simulink model "SDM"  (R2023b)
settings: Solver=FixedStepAuto  StartTime=0.0  StopTime=1  FixedStep=1/Fs  MaxStep=1/Fs  RelTol=1e-3
values from neighbouring files (symbols this model uses):
  f = Fs/2*linspace(0,1,NFFT/2+1)    [fft_plot.m]
undefined symbols (not defined in the file or in its folder): a1, a2, AAA, b1, b2, Fs, noise_pow1, noise_pow2
libraries: simulink x2
settings Model: Creator=mp3907  LastModifiedBy=mpolj
settings SolverCC: AlgebraicLoopSolver=TrustRegion
settings DataIOCC: ReturnWorkspaceOutputs=off
settings DebuggingCC: UnconnectedInputMsg=warning  UnconnectedOutputMsg=warning  UnconnectedLineMsg=warning  ArithmeticOperatorsInVariantConditions=warning
settings ModelReferenceCC: EnableRefExpFcnMdlSchedulingChecks=on
settings SFSimCC: CustomCodeUndefinedFunction=UseInterfaceOnly

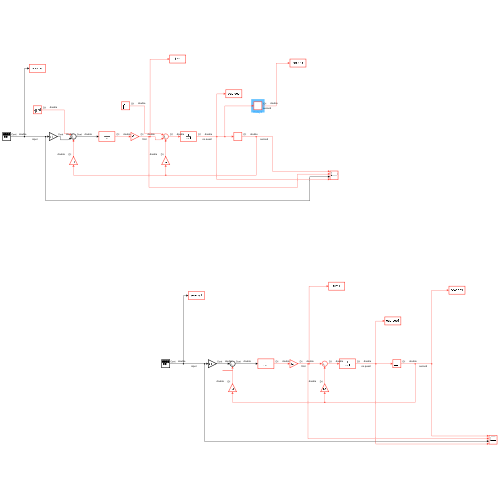
[thumbnail: Simulink's stored preview of the top-level diagram]
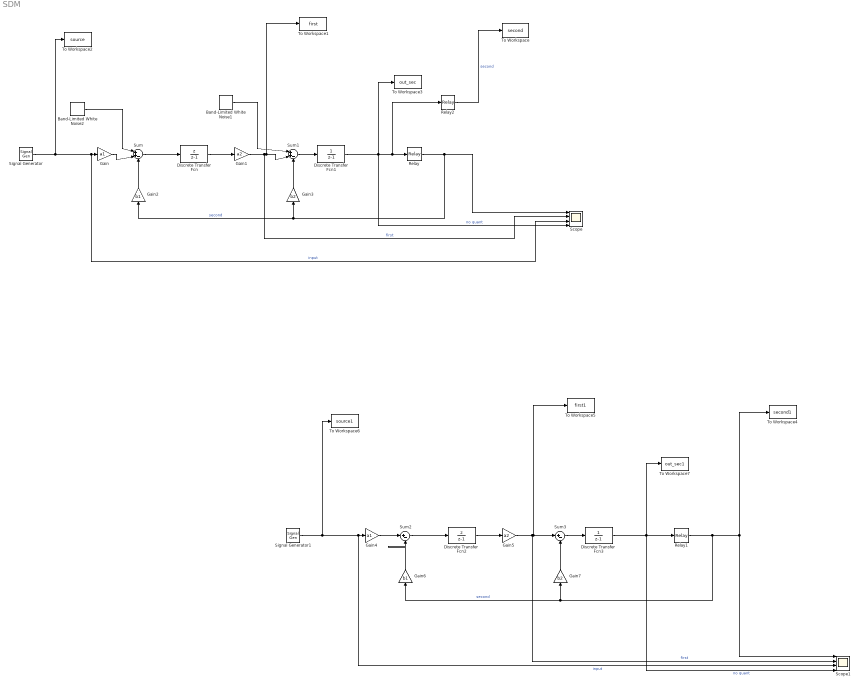
== system SDM ==
  Band-Limited White Noise1 : simulink/Sources/Band-Limited White Noise  Cov=[noise_pow2]  Ts=1/Fs  seed=[2341]
  Band-Limited White Noise2 : simulink/Sources/Band-Limited White Noise  Cov=[noise_pow1]  Ts=1/Fs  seed=[2341]
  Discrete Transfer Fcn : DiscreteTransferFcn  Numerator=[1 0]  Denominator=[1 -1]
  Discrete Transfer Fcn1 : DiscreteTransferFcn  Denominator=[1 -1]
  Discrete Transfer Fcn2 : DiscreteTransferFcn  Numerator=[1 0]  Denominator=[1 -1]
  Discrete Transfer Fcn3 : DiscreteTransferFcn  Denominator=[1 -1]
  Gain : Gain  Gain=a1
  Gain1 : Gain  Gain=a2
  Gain2 : Gain  Gain=b1
  Gain3 : Gain  Gain=b2
  Gain4 : Gain  Gain=a1
  Gain5 : Gain  Gain=a2
  Gain6 : Gain  Gain=b1
  Gain7 : Gain  Gain=b2
  Relay : Relay  OnSwitchValue=0  OffSwitchValue=0  OffOutputValue=-1
  Relay1 : Relay  OnSwitchValue=0  OffSwitchValue=0  OffOutputValue=-1
  Relay2 : Relay  OnSwitchValue=0  OffSwitchValue=0  OffOutputValue=-1
  Scope : Scope  NumInputPorts=4
  Scope1 : Scope  NumInputPorts=4
  Signal Generator : SignalGenerator  Amplitude=AAA  Frequency=f
  Signal Generator1 : SignalGenerator  Amplitude=AAA  Frequency=f
  Sum : Sum  Inputs=|++-
  Sum1 : Sum  Inputs=|++-
  Sum2 : Sum  Inputs=|+-
  Sum3 : Sum  Inputs=|+-
  To Workspace : ToWorkspace  VariableName=second  SaveFormat=Timeseries  SampleTime=-1
  To Workspace1 : ToWorkspace  VariableName=first  SaveFormat=Timeseries  SampleTime=-1
  To Workspace2 : ToWorkspace  VariableName=source  SaveFormat=Timeseries  SampleTime=-1
  To Workspace3 : ToWorkspace  VariableName=out_sec  SaveFormat=Timeseries  SampleTime=-1
  To Workspace4 : ToWorkspace  VariableName=second1  SaveFormat=Timeseries  SampleTime=-1
  To Workspace5 : ToWorkspace  VariableName=first1  SaveFormat=Timeseries  SampleTime=-1
  To Workspace6 : ToWorkspace  VariableName=source1  SaveFormat=Timeseries  SampleTime=-1
  To Workspace7 : ToWorkspace  VariableName=out_sec1  SaveFormat=Timeseries  SampleTime=-1
  wires:
  Discrete Transfer Fcn/1 -> Gain1/1
  Gain/1 -> Sum/2
  Gain2/1 -> Sum/3
  Sum/1 -> Discrete Transfer Fcn/1
  Gain1/1 -> Scope/2, Sum1/2, To Workspace1/1  "first"
  Sum1/1 -> Discrete Transfer Fcn1/1
  Gain3/1 -> Sum1/3
  Relay/1 -> Scope/1, Gain2/1, Gain3/1  "second"
  Signal Generator/1 -> To Workspace2/1, Scope/3, Gain/1  "input"
  Discrete Transfer Fcn1/1 -> To Workspace3/1, Relay2/1, Relay/1, Scope/4  "no quant"
  Band-Limited White Noise2/1 -> Sum/1
  Band-Limited White Noise1/1 -> Sum1/1
  Sum3/1 -> Discrete Transfer Fcn3/1
  Sum2/1 -> Discrete Transfer Fcn2/1
  Gain5/1 -> Scope1/2, Sum3/1, To Workspace5/1  "first"
  Discrete Transfer Fcn3/1 -> To Workspace7/1, Relay1/1, Scope1/4  "no quant"
  Gain6/1 -> Sum2/2
  Discrete Transfer Fcn2/1 -> Gain5/1
  Gain4/1 -> Sum2/1
  Signal Generator1/1 -> To Workspace6/1, Scope1/3, Gain4/1  "input"
  Relay1/1 -> To Workspace4/1, Scope1/1, Gain6/1, Gain7/1  "second"
  Gain7/1 -> Sum3/2
  Relay2/1 -> To Workspace/1  "second"
